simulink model "Hamish_Sams_EEE6205_02c"  (Simulink 9.2)
settings: Solver=VariableStepDiscrete  StartTime=0.0  StopTime=0.06  RelTol=1e-3
InitFcn:
  | Ts=1e-7
  | fo=70;
  | fc=5000;
  | Rout=10;
  | Lout=5e-3;
  | AmplitudeIn=0.881;
libraries: powerlib x9, simulink x1
settings Model: Creator=hamishsams  LastModifiedBy=hamishsams
settings DataIOCC: LimitDataPoints=off  SaveFormat=Dataset  SignalLoggingSaveFormat=Dataset
settings OptimizationCC: LifeSpan=auto
settings DebuggingCC: UnderspecifiedInitializationDetection=Simplified  MergeDetectMultiDrivingBlocksExec=error  FcnCallInpInsideContextMsg=error  StateNameClashWarn=none  SFUnexpectedBacktrackingDiag=error  SFNoUnconditionalDefaultTransitionDiag=error  SFExecutionAtInitializationDiag=warning
settings HardwareCC: ProdBitPerPointer=64  ProdBitPerSizeT=64  ProdBitPerPtrDiffT=64  ProdLargestAtomicFloat=Float  ProdIntDivRoundTo=Zero  ProdEndianess=LittleEndian  ProdWordSize=64  ProdHWDeviceType=Intel->x86-64 (Windows64)
settings ModelReferenceCC: PropagateSignalLabelsOutOfModel=on
settings SFSimCC: SimUseLocalCustomCode=on
settings RTWCC: RTWUseLocalCustomCode=on
settings CodeAppCC: StateflowObjectComments=off
settings GRTTargetCC: TargetLangStandard=C99 (ISO)  GeneratePreprocessorConditionals=Use local settings  CombineOutputUpdateFcns=on  GRTInterface=off
settings ConfigComp: CovMetricSettings=dwe  CovHtmlReporting=off  CovSaveCumulativeToWorkspaceVar=off  CovSaveSingleToWorkspaceVar=off  CovExternalEMLEnable=on

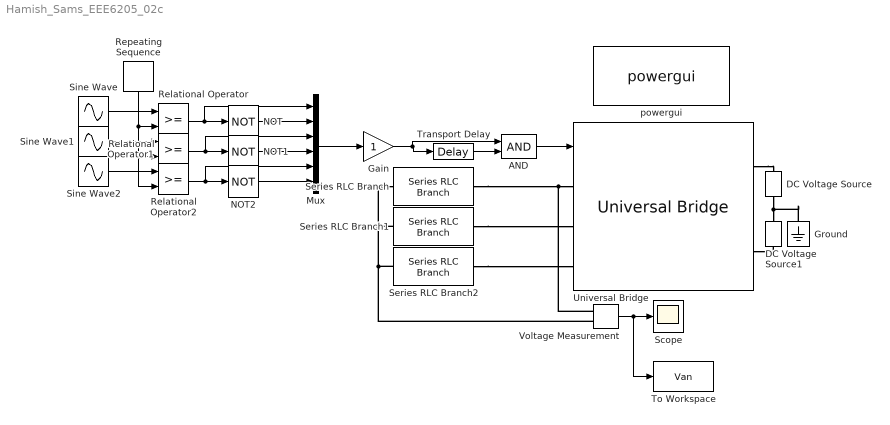
== system Hamish_Sams_EEE6205_02c ==
  AND : Logic  IconShape=distinctive  AllPortsSameDT=off  OutDataTypeStr=boolean
  DC Voltage Source : powerlib/Electrical Sources/DC Voltage Source  Amplitude=250  Measurements=None
  DC Voltage Source1 : powerlib/Electrical Sources/DC Voltage Source  Amplitude=250  Measurements=None
  Gain : Gain  OutDataTypeStr=double
  Ground : powerlib/Elements/Ground  LConnTagsString=a
  Mux : Mux  Inputs=6
  NOT : Logic  Operator=NOT  IconShape=distinctive  AllPortsSameDT=off  OutDataTypeStr=boolean
  NOT1 : Logic  Operator=NOT  IconShape=distinctive  AllPortsSameDT=off  OutDataTypeStr=boolean
  NOT2 : Logic  Operator=NOT  IconShape=distinctive  AllPortsSameDT=off  OutDataTypeStr=boolean
  Relational Operator : RelationalOperator  OutDataTypeStr=boolean  RndMeth=Simplest
  Relational Operator1 : RelationalOperator  OutDataTypeStr=boolean  RndMeth=Simplest
  Relational Operator2 : RelationalOperator  OutDataTypeStr=boolean  RndMeth=Simplest
  Repeating Sequence : simulink/Sources/Repeating Sequence  rep_seq_t=[0 1/(200*fo)]  rep_seq_y=[-1 1]
  Scope : Scope
  Series RLC Branch : powerlib/Elements/Series RLC Branch  LConnTagsString=__new0  RConnTagsString=__new0  BranchType=RL  Resistance=Rout  Inductance=Lout  SetiL0=off  InitialCurrent=0  Capacitance=1e-6  Setx0=off  InitialVoltage=0  Measurements=None
  Series RLC Branch1 : powerlib/Elements/Series RLC Branch  LConnTagsString=__new0  RConnTagsString=__new0  BranchType=RL  Resistance=Rout  Inductance=Lout  SetiL0=off  InitialCurrent=0  Capacitance=1e-6  Setx0=off  InitialVoltage=0  Measurements=None
  Series RLC Branch2 : powerlib/Elements/Series RLC Branch  LConnTagsString=__new0  RConnTagsString=__new0  BranchType=RL  Resistance=Rout  Inductance=Lout  SetiL0=off  InitialCurrent=0  Capacitance=1e-6  Setx0=off  InitialVoltage=0  Measurements=None
  Sine Wave : Sin  Amplitude=AmplitudeIn  Frequency=2*pi*fo  SampleTime=0
  Sine Wave1 : Sin  Amplitude=AmplitudeIn  Frequency=2*pi*fo  Phase=2*pi/3  SampleTime=0
  Sine Wave2 : Sin  Amplitude=AmplitudeIn  Frequency=2*pi*fo  Phase=4*pi/3  SampleTime=0
  To Workspace : ToWorkspace  VariableName=Van  SaveFormat=Structure With Time  SampleTime=-1
  Transport Delay : TransportDelay  DelayTime=3e-6
  Universal Bridge : powerlib/Power Electronics/Universal Bridge  Arms=3  SnubberResistance=1e5  SnubberCapacitance=inf  Device=IGBT / Diodes  Ron=1e-6  Lon=0  ForwardVoltages="[  0  0.7  ]"  ForwardVoltage=0  GTOparameters=[ 10e-6 , 20e-6 ]  IGBTparameters=[ 1e-6 , 2e-6 ]  Measurements=Device currents  Measurements_2=None  converterType=Rectifier
  Voltage Measurement : powerlib/Measurements/Voltage Measurement  PhasorSimulation=off  OutputType=Complex  PSBequivalent=0
  powergui : powerlib/powergui  Priority=1  SimulationMode=Discrete  SampleTime=1e-6  frequency=60  Iterations=50  frequencyindice=0  Pbase=100e6  ErrMax=1e-4  UnitsV=kV  UnitsW=MW  buscounter=0  FunctionMessages=off  echomessages=off  EnableUseOfTLC=off  CurrentSourceSwitches=off  DisableSnubberDevices=off  DisableRonSwitches=off  DisableVfSwitches=off  DisplayEquations=off  SolverType=Tustin  Interpol=off  ExternalGateDelay=off  methode=off  Ts=100  x0status=blocks  SPID=on  SwTol=0  HookPort=off  RestoreLinks=warning  ResistiveCurrentMeasurement=off  Frange=[0:2:500]  Ylog=off  Xlog=on  ShowGrid=off  save=off  variable=ZData  structure=0  ZoomFFT=off  StartTime=0.0  cycles=1  DisplayStyle=1  fundamental=60  FreqAxis=off  MaxFrequency=1000  frequencyindicesteady=1  RmsSteady=1  display=off
  wires:
  Repeating Sequence/1 -> Relational Operator/2, Relational Operator1/2, Relational Operator2/2
  Sine Wave2/1 -> Relational Operator2/1
  Sine Wave1/1 -> Relational Operator1/1
  Sine Wave/1 -> Relational Operator/1
  Relational Operator/1 -> Mux/1, NOT/1
  Relational Operator1/1 -> NOT1/1, Mux/3
  Relational Operator2/1 -> Mux/5, NOT2/1
  Voltage Measurement/1 -> To Workspace/1, Scope/1
  Transport Delay/1 -> AND/2
  NOT/1 -> Mux/2
  NOT1/1 -> Mux/4
  NOT2/1 -> Mux/6
  AND/1 -> Universal Bridge/1
  Mux/1 -> Gain/1
  Gain/1 -> AND/1, Transport Delay/1
  connections:
  Voltage Measurement/LConn1 -- Series RLC Branch/LConn1 -- Universal Bridge/LConn1
  Series RLC Branch1/LConn1 -- Universal Bridge/LConn2
  Series RLC Branch2/LConn1 -- Universal Bridge/LConn3
  Series RLC Branch2/RConn1 -- Series RLC Branch1/RConn1 -- Series RLC Branch/RConn1 -- Voltage Measurement/LConn2
  DC Voltage Source/LConn1 -- Ground/LConn1 -- DC Voltage Source1/RConn1
  Universal Bridge/RConn2 -- DC Voltage Source1/LConn1
  Universal Bridge/RConn1 -- DC Voltage Source/RConn1
